simulink model "test_lightsensors"  (Simulink 5.0)
settings: Solver=ode5  StartTime=0.0  StopTime=10.0  FixedStep=0.01  RelTol=1e-3
undefined symbols (not defined in the file): sigbuilder_block
CloseFcn:
  | rtwprivate ssgencode ModelCloseRequest test_onoffbutton
settings Model: Creator=riccardo  LastModifiedBy=riccardo  ExtModeMexFile=no_ext_comm  ExtModeAutoUpdateStatusClock=off  ConsistencyChecking=error  ArrayBoundsChecking=error  RTWSystemTargetFile=ErikaEducational.tlc  RTWTemplateMakefile=ErikaEducational.tmf  RTWGenerateCodeOnly=on  RTWOptions="-aDOWNLCOMM=\"firmdl\" -aDebugLcd=0 -aDownloadToRobot=0 -aERIKABASE=\"/home/riccardo/ErikaEducational/erika\" -aEnforceIntegerDowncast=1 -aFoldNonRolledExpr=1 -aForceParamTrailComments=0 -aGenerateComments=1 -aGenerateReport=0 -aH8RTWLIBDIR=\"/home/riccardo/gencod/lib\" -aIncDataTypeInIds=0 -aIncHierarchyInIds=0 -aInlineInvariantSignals=0 -aInlinedPrmAccess=\"Literals\" -aLEGOTOWERDEVICE=\"/dev/usb/lego0\" -aLocalBlockOutputs=0 -aMaxRTWIdLen=31 -aPrefixModelToSubsysFcnNames=1 -aRTNONFINITE=0 -aRTWVerbose=1 -aRollThreshold=5 -aShowEliminatedStatements=0 -aTaskCF=0 -aUSECUSTCOMM=0 -aUseERT=0 -aVarProcTask=0"

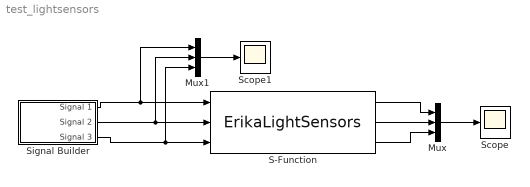
== system test_lightsensors ==
  Mux : Mux  Inputs=3
  Mux1 : Mux  Inputs=3
  S-Function : S-Function  FunctionName=ErikaLightSensors  Parameters=7 1 9
  Scope : Scope
  Scope1 : Scope
  Signal Builder : Subsystem  Tag=STV Subsys  StartFcn=sigbuilder_block('start');  StopFcn=sigbuilder_block('stop');  ClipboardFcn=sigbuilder_block('clipboard');  mask(Sigbuilder block){}
      mask help: Sigbuilder GUI
      mask init:
      | if ~strcmp(get_param(bdroot(gcb),'SimulationStatus'),'stopped') tuvar = sigbuilder_block('maskInit'); end
      settings: CopyFcn=sigbuilder_block('copy');  DeleteFcn=sigbuilder_block('delete');  ModelCloseFcn=sigbuilder_block('modelClose');  PreSaveFcn=sigbuilder_block('preSave');  NameChangeFcn=sigbuilder_block('namechange');  OpenFcn=sigbuilder_block('open',[49.92 52.8 520.32 400.32 ]);  CloseFcn=sigbuilder_block('close');
      mask Display: plot(0,0,100,100,[10,10,40,40,10],[80,20,20,80,80],[40,10],[50,50], [40,27,10],[65,72,56],[40,25,25,10],[28,28,43,43]);
  wires:
  S-Function/1 -> Mux/1
  S-Function/2 -> Mux/2
  S-Function/3 -> Mux/3
  Mux/1 -> Scope/1
  Signal Builder/1(Signal 1) -> Mux1/1, S-Function/1
  Signal Builder/2(Signal 2) -> S-Function/2, Mux1/2
  Signal Builder/3(Signal 3) -> S-Function/3, Mux1/3
  Mux1/1 -> Scope1/1

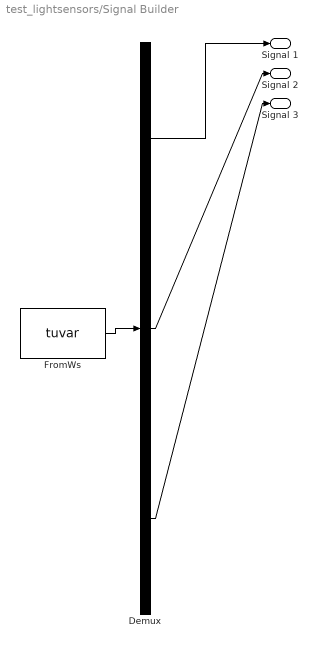
== system test_lightsensors/Signal Builder ==
  Demux : Demux  Tag=STV Demux  Outputs=3
  FromWs : FromWorkspace  Tag=STV FromWs  VariableName=tuvar  SampleTime=0  SigBuilderData=DataTag0
      SigBuilderData=|
      | channels(1).label = 'Signal 1'
      | channels(1).allXData = {[0 4 4 6 6 10]}
      | channels(1).allYData = {[3.64 3.64 14.05 14.05 50.6 50.6]}
      | channels(2).label = 'Signal 2'
      | channels(2).allXData = {[0 4 4 6 6 10]}
      | channels(2).allYData = {[21.8 21.8 43.5 43.5 33.5 33.5]}
      | channels(3).label = 'Signal 3'
      | channels(3).allXData = {[0 4 4 6 6 10]}
      | channels(3).allYData = {[11.6 11.6 5.46 5.46 14.9 14.9]}
      | dataSet.timeRange = [0 10]
      | dataSet.name = 'Group 1'
  Signal 1 : Outport  Tag=STV Outport
  Signal 2 : Outport  Tag=STV Outport  Port=2
  Signal 3 : Outport  Tag=STV Outport  Port=3
  wires:
  Demux/1 -> Signal 1/1
  FromWs/1 -> Demux/1
  Demux/2 -> Signal 2/1
  Demux/3 -> Signal 3/1
